simulink model "MyModel"  (R2020b)
settings: Solver=VariableStepAuto  StartTime=0.0  StopTime=50  RelTol=1e-3
undefined symbols (not defined in the file or in its folder): InnerLoop
libraries: simulink x6
settings Model: Creator=Aurelien_Julien  LastModifiedBy=Aurelien_Julien

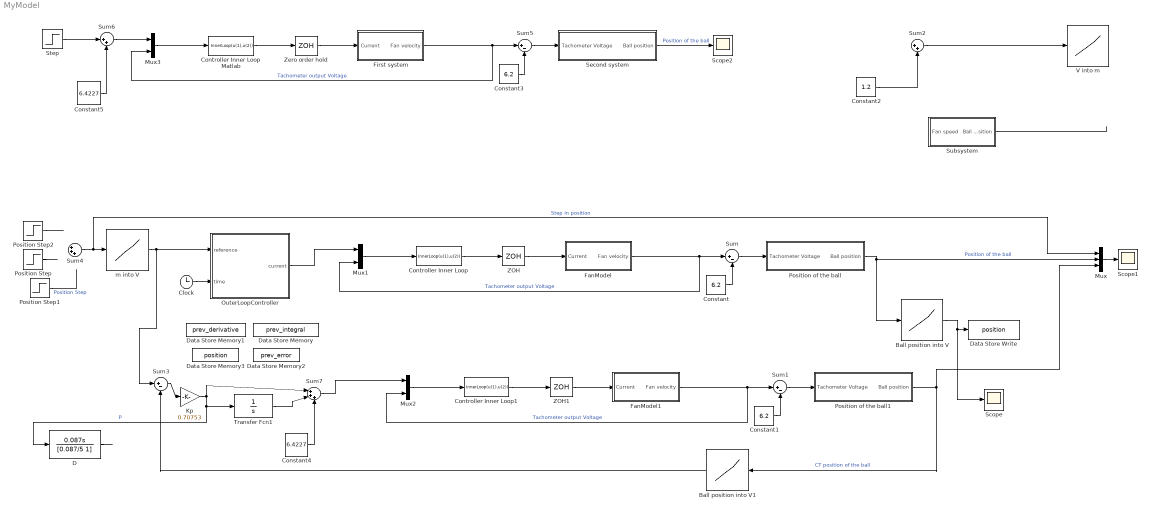
== system MyModel ==
  Ball position into V : Lookup_n-D  NumberOfTableDimensions=1  BreakpointsForDimension1=[0 15 60 97.5 117.5 125 127.5 132 135 138 142 148 152 160 167.5 180]/100  Table=[1.2 1.4 1.8 2.4 2.5 2.75 3.1 3.5 3.9 4.5 5.2 5.6 5.7 6.3 6.7 7.32]  InternalRulePriority=Speed  RndMeth=Simplest  InputSameDT=on
  Ball position into V1 : Lookup_n-D  NumberOfTableDimensions=1  BreakpointsForDimension1=[0 15 60 97.5 117.5 125 127.5 132 135 138 142 148 152 160 167.5 180]/100  Table=[1.2 1.4 1.8 2.4 2.5 2.75 3.1 3.5 3.9 4.5 5.2 5.6 5.7 6.3 6.7 7.32]  InternalRulePriority=Speed  RndMeth=Simplest  InputSameDT=on
  Clock : Clock
  Constant : Constant  Value=6.2
  Constant1 : Constant  Value=6.2
  Constant2 : Constant  Value=1.2
  Constant3 : Constant  Value=6.2
  Constant4 : Constant  Value=6.4227
  Constant5 : Constant  Value=6.4227
  Controller Inner Loop : MATLABFcn  MATLABFcn=InnerLoop(u(1),u(2))  OutputDimensions=1
  Controller Inner Loop Matlab : MATLABFcn  MATLABFcn=InnerLoop(u(1),u(2))  OutputDimensions=1
  Controller Inner Loop1 : MATLABFcn  MATLABFcn=InnerLoop(u(1),u(2))  OutputDimensions=1
  D : TransferFcn  Numerator=[0.087 0]  Denominator=[0.087/5 1]
  Data Store Memory : DataStoreMemory  DataStoreName=prev_integral  ReadBeforeWriteMsg=warning  WriteAfterWriteMsg=warning  WriteAfterReadMsg=warning  ShowAdditionalParam=off  OutDataTypeStr=double
  Data Store Memory1 : DataStoreMemory  DataStoreName=prev_derivative  ReadBeforeWriteMsg=warning  WriteAfterWriteMsg=warning  WriteAfterReadMsg=warning  ShowAdditionalParam=off  OutDataTypeStr=double
  Data Store Memory2 : DataStoreMemory  DataStoreName=prev_error  ReadBeforeWriteMsg=warning  WriteAfterWriteMsg=warning  WriteAfterReadMsg=warning  ShowAdditionalParam=off  OutDataTypeStr=double
  Data Store Memory3 : DataStoreMemory  DataStoreName=position  ReadBeforeWriteMsg=warning  WriteAfterWriteMsg=warning  WriteAfterReadMsg=warning  ShowAdditionalParam=off  OutDataTypeStr=double
  Data Store Write : DataStoreWrite  DataStoreName=position  SampleTime=0.01
  FanModel : Subsystem
  FanModel1 : Subsystem
  First system : Subsystem
  Kp : Gain  Gain=0.70753
  Mux : Mux  Inputs=3
  Mux1 : Mux  Inputs=2
  Mux2 : Mux  Inputs=2
  Mux3 : Mux  Inputs=2
  OuterLoopController : MATLAB Function  TreatAsAtomicUnit=on  SystemSampleTime=0.01
  Position Step : Step  Time=20  Before=1.2  After=1.6  SampleTime=0
  Position Step1 : Step  Time=30  After=-0.3  SampleTime=0
  Position Step2 : Step  Time=5  After=0.8  SampleTime=0
  Position of the ball : Subsystem
  Position of the ball1 : Subsystem
  Scope : Scope
  Scope1 : Scope
  Scope2 : Scope
  Second system : Subsystem
  Step : Step  SampleTime=0
  Subsystem : Subsystem
  Sum{,1,3,5} (4 alike) : Sum  Inputs=|+-
  Sum2 : Sum  Inputs=|++
  Sum4 : Sum  Inputs=|+++
  Sum6 : Sum  Inputs=|++
  Sum7 : Sum  Inputs=|+++
  Transfer Fcn1 : TransferFcn  Denominator=[1 0]
  V into m : Lookup_n-D  NumberOfTableDimensions=1  BreakpointsForDimension1=[1.2 1.4 1.8 2.4 2.5 2.75 3.1 3.5 3.9 4.5 5.2 5.6 5.7 6.3 6.7 7.32]  Table=[0 15 60 97.5 117.5 125 127.5 132 135 138 142 148 152 160 167.5 180]/100  InternalRulePriority=Speed  RndMeth=Simplest  InputSameDT=on
  ZOH : ZeroOrderHold  SampleTime=0.01
  ZOH1 : ZeroOrderHold  SampleTime=0.01
  Zero order hold : ZeroOrderHold  SampleTime=0.01
  m into V : Lookup_n-D  NumberOfTableDimensions=1  BreakpointsForDimension1=[0 15 60 97.5 117.5 125 127.5 132 135 138 142 148 152 160 167.5 180]/100  Table=[1.2 1.4 1.8 2.4 2.5 2.75 3.1 3.5 3.9 4.5 5.2 5.6 5.7 6.3 6.7 7.32]  InternalRulePriority=Speed  RndMeth=Simplest  InputSameDT=on
  wires:
  Subsystem/1(Ball Position) -> ?
  Mux1/1 -> Controller Inner Loop/1
  FanModel/1(Fan velocity) -> Sum/1, Mux1/2  "Tachometer output Voltage"
  ZOH/1 -> FanModel/1(Current)
  Controller Inner Loop/1 -> ZOH/1
  Mux/1 -> Scope1/1
  Sum/1 -> Position of the ball/1(Tachometer Voltage)
  Constant/1 -> Sum/2
  Position of the ball/1(Ball position) -> Mux/2, Ball position into V/1  "Position of the ball"
  Sum2/1 -> V into m/1
  Constant2/1 -> Sum2/2
  Sum4/1 -> Mux/1, m into V/1  "Step in position"
  Ball position into V/1 -> Scope/1, Data Store Write/1
  Kp/1 -> Transfer Fcn1/1, D/1, Sum7/1  "P"
  Constant4/1 -> Sum7/3
  Position Step1/1 -> ?  "Position Step"
  D/1 -> ?
  Clock/1 -> OuterLoopController/2(time)
  OuterLoopController/1(current) -> Mux1/1
  m into V/1 -> Sum3/1, OuterLoopController/1(reference)
  Position Step/1 -> ?
  Position Step2/1 -> ?
  Sum1/1 -> Position of the ball1/1(Tachometer Voltage)
  Constant1/1 -> Sum1/2
  FanModel1/1(Fan velocity) -> Sum1/1, Mux2/2  "Tachometer output Voltage"
  Controller Inner Loop1/1 -> ZOH1/1
  ZOH1/1 -> FanModel1/1(Current)
  Sum7/1 -> Mux2/1
  Mux2/1 -> Controller Inner Loop1/1
  Position of the ball1/1(Ball position) -> Mux/3, Ball position into V1/1  "CT position of the ball"
  Sum3/1 -> Kp/1
  Ball position into V1/1 -> Sum3/2
  Transfer Fcn1/1 -> Sum7/2
  Constant3/1 -> Sum5/2
  Sum5/1 -> Second system/1(Tachometer Voltage)
  First system/1(Fan velocity) -> Sum5/1, Mux3/2  "Tachometer output Voltage"
  Zero order hold/1 -> First system/1(Current)
  Controller Inner Loop Matlab/1 -> Zero order hold/1
  Step/1 -> Sum6/1
  Mux3/1 -> Controller Inner Loop Matlab/1
  Second system/1(Ball position) -> Scope2/1  "Position of the ball"
  Constant5/1 -> Sum6/2
  Sum6/1 -> Mux3/1

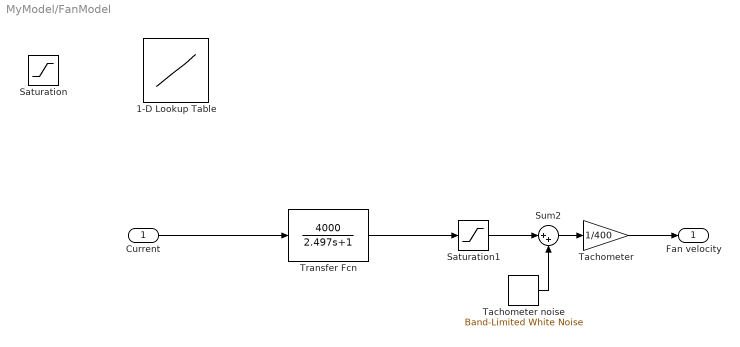
== system MyModel/FanModel ==
  Current : Inport
  1-D Lookup Table : Lookup_n-D  NumberOfTableDimensions=1  BreakpointsForDimension1=[-4 -1 0 1 2 2.5 4]  Table=[-1450 -1300 0 1600 2800 3600 3800]  InternalRulePriority=Speed  RndMeth=Simplest  InputSameDT=on
  Saturation : Saturate  UpperLimit=7  LowerLimit=-7
  Saturation1 : Saturate  UpperLimit=9.6*400  LowerLimit=-3.6*400
  Sum2 : Sum  Inputs=|++
  Tachometer : Gain  Gain=1/400
  Tachometer noise : simulink/Sources/Band-Limited White Noise  Cov=[0.1]  Ts=0.01  seed=[23341]
  Transfer Fcn : TransferFcn  Numerator=[4000]  Denominator=[2.497 1]
  Fan velocity : Outport
  wires:
  Transfer Fcn/1 -> Saturation1/1
  Current/1 -> Transfer Fcn/1
  Tachometer/1 -> Fan velocity/1
  Tachometer noise/1 -> Sum2/2
  Saturation1/1 -> Sum2/1
  Sum2/1 -> Tachometer/1

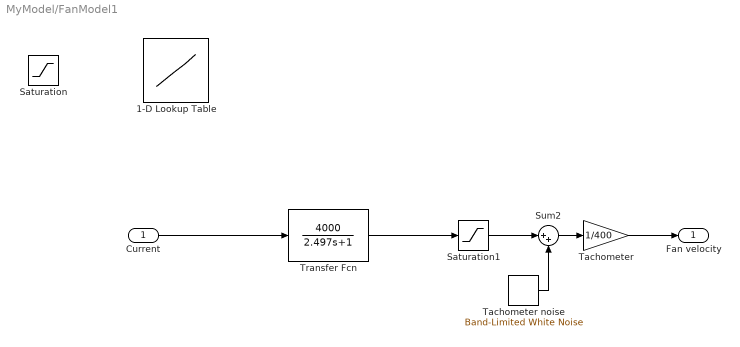
== system MyModel/FanModel1 ==
  Current : Inport
  1-D Lookup Table : Lookup_n-D  NumberOfTableDimensions=1  BreakpointsForDimension1=[-4 -1 0 1 2 2.5 4]  Table=[-1450 -1300 0 1600 2800 3600 3800]  InternalRulePriority=Speed  RndMeth=Simplest  InputSameDT=on
  Saturation : Saturate  UpperLimit=7  LowerLimit=-7
  Saturation1 : Saturate  UpperLimit=9.6*400  LowerLimit=-3.6*400
  Sum2 : Sum  Inputs=|++
  Tachometer : Gain  Gain=1/400
  Tachometer noise : simulink/Sources/Band-Limited White Noise  Cov=[0.1]  Ts=0.01  seed=[23341]
  Transfer Fcn : TransferFcn  Numerator=[4000]  Denominator=[2.497 1]
  Fan velocity : Outport
  wires:
  Transfer Fcn/1 -> Saturation1/1
  Current/1 -> Transfer Fcn/1
  Tachometer/1 -> Fan velocity/1
  Tachometer noise/1 -> Sum2/2
  Saturation1/1 -> Sum2/1
  Sum2/1 -> Tachometer/1

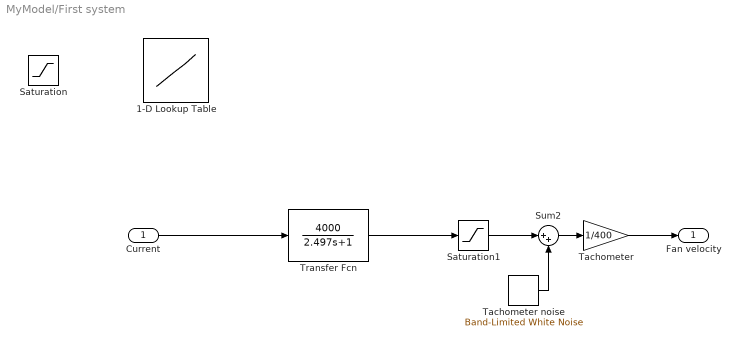
== system MyModel/First system ==
  Current : Inport
  1-D Lookup Table : Lookup_n-D  NumberOfTableDimensions=1  BreakpointsForDimension1=[-4 -1 0 1 2 2.5 4]  Table=[-1450 -1300 0 1600 2800 3600 3800]  InternalRulePriority=Speed  RndMeth=Simplest  InputSameDT=on
  Saturation : Saturate  UpperLimit=7  LowerLimit=-7
  Saturation1 : Saturate  UpperLimit=9.6*400  LowerLimit=-3.6*400
  Sum2 : Sum  Inputs=|++
  Tachometer : Gain  Gain=1/400
  Tachometer noise : simulink/Sources/Band-Limited White Noise  Cov=[0.1]  Ts=0.01  seed=[23341]
  Transfer Fcn : TransferFcn  Numerator=[4000]  Denominator=[2.497 1]
  Fan velocity : Outport
  wires:
  Transfer Fcn/1 -> Saturation1/1
  Current/1 -> Transfer Fcn/1
  Tachometer/1 -> Fan velocity/1
  Tachometer noise/1 -> Sum2/2
  Saturation1/1 -> Sum2/1
  Sum2/1 -> Tachometer/1

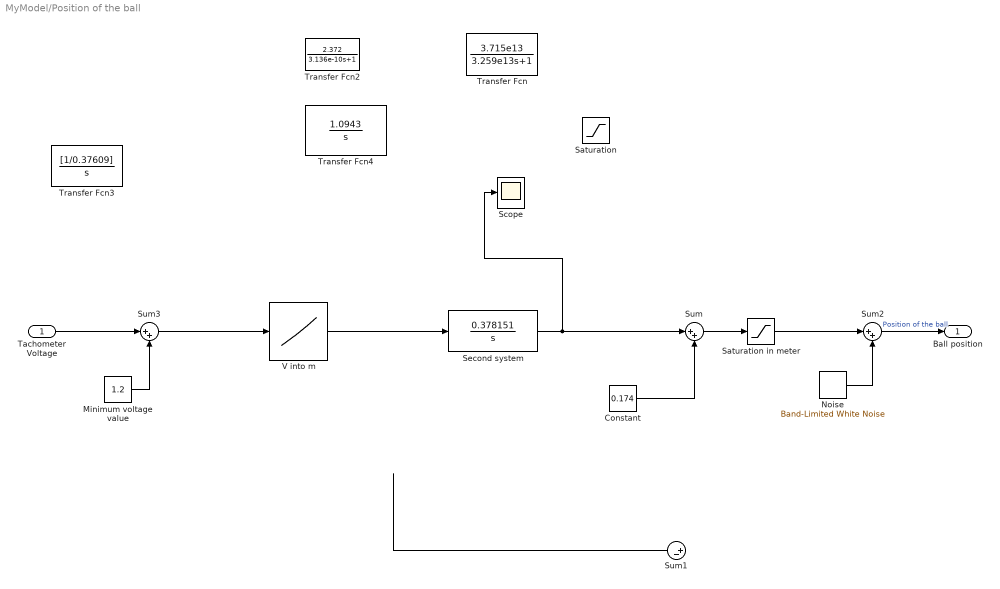
== system MyModel/Position of the ball ==
  Tachometer Voltage : Inport
  Constant : Constant  Value=0.174
  Minimum voltage value : Constant  Value=1.2
  Noise : simulink/Sources/Band-Limited White Noise  Cov=[0.0000001]  Ts=0.01  seed=[23341]
  Saturation : Saturate  UpperLimit=6.12  LowerLimit=0
  Saturation in meter : Saturate  UpperLimit=1.8  LowerLimit=0
  Scope : Scope
  Second system : TransferFcn  Numerator=[0.378151]  Denominator=[1 0]
  Sum : Sum  Inputs=|++
  Sum1 : Sum  Inputs=|+-
  Sum2 : Sum  Inputs=|++
  Sum3 : Sum  Inputs=|++
  Transfer Fcn : TransferFcn  Numerator=[3.715e13]  Denominator=[3.259e13 1]
  Transfer Fcn2 : TransferFcn  Numerator=[2.372]  Denominator=[3.136e-10 1]
  Transfer Fcn3 : TransferFcn  Numerator=[1/0.37609]  Denominator=[1 0]
  Transfer Fcn4 : TransferFcn  Numerator=[1.0943]  Denominator=[1 0]
  V into m : Lookup_n-D  NumberOfTableDimensions=1  BreakpointsForDimension1=[1.2 1.4 1.8 2.4 2.5 2.75 3.1 3.5 3.9 4.5 5.2 5.6 5.7 6.3 6.7 7.32]  Table=[0 15 60 97.5 117.5 125 127.5 132 135 138 142 148 152 160 167.5 180]/100  InternalRulePriority=Speed  RndMeth=Simplest  InputSameDT=on
  Ball position : Outport
  wires:
  Constant/1 -> Sum/2
  Sum/1 -> Saturation in meter/1
  Sum1/1 -> ?
  Minimum voltage value/1 -> Sum3/2
  Second system/1 -> Scope/1, Sum/1
  Saturation in meter/1 -> Sum2/1
  V into m/1 -> Second system/1
  Tachometer Voltage/1 -> Sum3/1
  Sum3/1 -> V into m/1
  Noise/1 -> Sum2/2
  Sum2/1 -> Ball position/1  "Position of the ball"

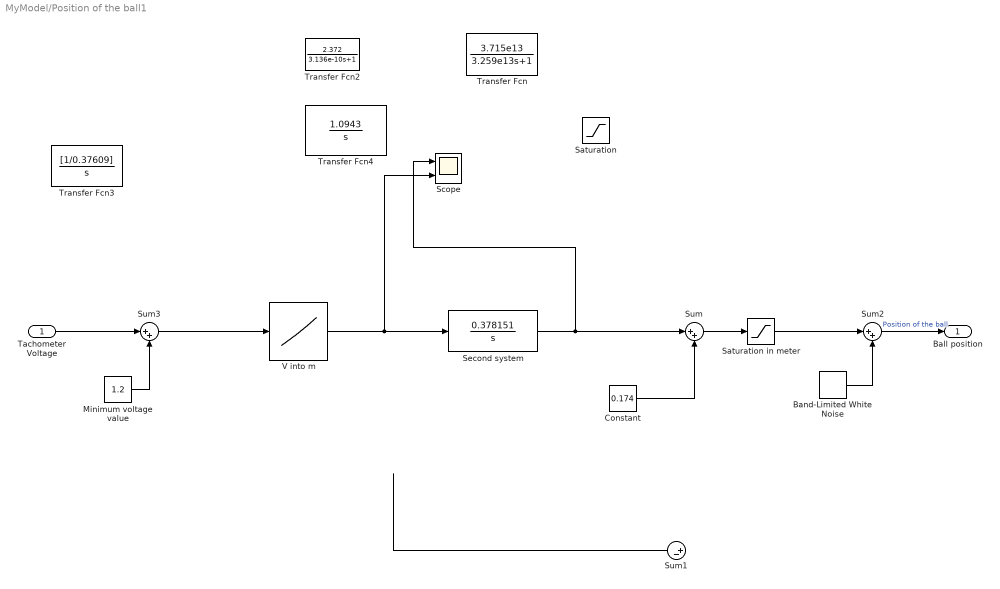
== system MyModel/Position of the ball1 ==
  Tachometer Voltage : Inport
  Band-Limited White Noise : simulink/Sources/Band-Limited White Noise  Cov=[0.0000001]  Ts=0.01  seed=[23341]
  Constant : Constant  Value=0.174
  Minimum voltage value : Constant  Value=1.2
  Saturation : Saturate  UpperLimit=6.12  LowerLimit=0
  Saturation in meter : Saturate  UpperLimit=1.8  LowerLimit=0
  Scope : Scope  NumInputPorts=2
  Second system : TransferFcn  Numerator=[0.378151]  Denominator=[1 0]
  Sum : Sum  Inputs=|++
  Sum1 : Sum  Inputs=|+-
  Sum2 : Sum  Inputs=|++
  Sum3 : Sum  Inputs=|++
  Transfer Fcn : TransferFcn  Numerator=[3.715e13]  Denominator=[3.259e13 1]
  Transfer Fcn2 : TransferFcn  Numerator=[2.372]  Denominator=[3.136e-10 1]
  Transfer Fcn3 : TransferFcn  Numerator=[1/0.37609]  Denominator=[1 0]
  Transfer Fcn4 : TransferFcn  Numerator=[1.0943]  Denominator=[1 0]
  V into m : Lookup_n-D  NumberOfTableDimensions=1  BreakpointsForDimension1=[1.2 1.4 1.8 2.4 2.5 2.75 3.1 3.5 3.9 4.5 5.2 5.6 5.7 6.3 6.7 7.32]  Table=[0 15 60 97.5 117.5 125 127.5 132 135 138 142 148 152 160 167.5 180]/100  InternalRulePriority=Speed  RndMeth=Simplest  InputSameDT=on
  Ball position : Outport
  wires:
  Constant/1 -> Sum/2
  Sum/1 -> Saturation in meter/1
  Sum1/1 -> ?
  Minimum voltage value/1 -> Sum3/2
  Second system/1 -> Scope/1, Sum/1
  Saturation in meter/1 -> Sum2/1
  V into m/1 -> Scope/2, Second system/1
  Tachometer Voltage/1 -> Sum3/1
  Sum3/1 -> V into m/1
  Band-Limited White Noise/1 -> Sum2/2
  Sum2/1 -> Ball position/1  "Position of the ball"

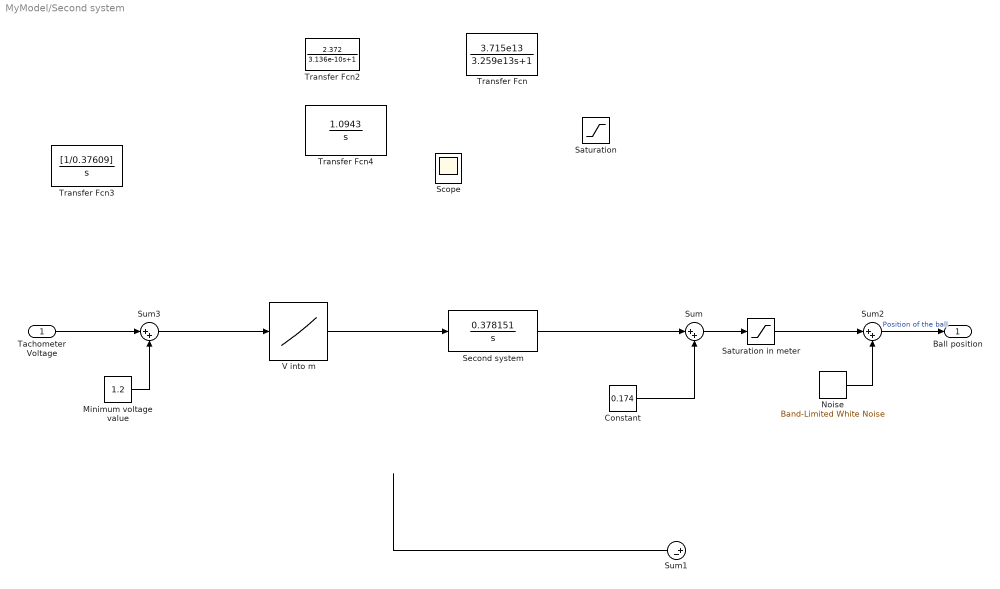
== system MyModel/Second system ==
  Tachometer Voltage : Inport
  Constant : Constant  Value=0.174
  Minimum voltage value : Constant  Value=1.2
  Noise : simulink/Sources/Band-Limited White Noise  Cov=[0.0000001]  Ts=0.01  seed=[23341]
  Saturation : Saturate  UpperLimit=6.12  LowerLimit=0
  Saturation in meter : Saturate  UpperLimit=1.8  LowerLimit=0
  Scope : Scope  NumInputPorts=2
  Second system : TransferFcn  Numerator=[0.378151]  Denominator=[1 0]
  Sum : Sum  Inputs=|++
  Sum1 : Sum  Inputs=|+-
  Sum2 : Sum  Inputs=|++
  Sum3 : Sum  Inputs=|++
  Transfer Fcn : TransferFcn  Numerator=[3.715e13]  Denominator=[3.259e13 1]
  Transfer Fcn2 : TransferFcn  Numerator=[2.372]  Denominator=[3.136e-10 1]
  Transfer Fcn3 : TransferFcn  Numerator=[1/0.37609]  Denominator=[1 0]
  Transfer Fcn4 : TransferFcn  Numerator=[1.0943]  Denominator=[1 0]
  V into m : Lookup_n-D  NumberOfTableDimensions=1  BreakpointsForDimension1=[1.2 1.4 1.8 2.4 2.5 2.75 3.1 3.5 3.9 4.5 5.2 5.6 5.7 6.3 6.7 7.32]  Table=[0 15 60 97.5 117.5 125 127.5 132 135 138 142 148 152 160 167.5 180]/100  InternalRulePriority=Speed  RndMeth=Simplest  InputSameDT=on
  Ball position : Outport
  wires:
  Constant/1 -> Sum/2
  Sum/1 -> Saturation in meter/1
  Sum1/1 -> ?
  Minimum voltage value/1 -> Sum3/2
  Second system/1 -> Sum/1
  Saturation in meter/1 -> Sum2/1
  V into m/1 -> Second system/1
  Tachometer Voltage/1 -> Sum3/1
  Sum3/1 -> V into m/1
  Noise/1 -> Sum2/2
  Sum2/1 -> Ball position/1  "Position of the ball"

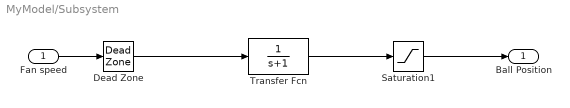
== system MyModel/Subsystem ==
  Fan speed : Inport
  Dead Zone : DeadZone  LowerValue=-11  UpperValue=6.25  SaturateOnIntegerOverflow=on
  Saturation1 : Saturate  UpperLimit=7.32  LowerLimit=1.2
  Transfer Fcn : TransferFcn  Denominator=[1 1]
  Ball Position : Outport
  wires:
  Fan speed/1 -> Dead Zone/1
  Dead Zone/1 -> Transfer Fcn/1
  Transfer Fcn/1 -> Saturation1/1
  Saturation1/1 -> Ball Position/1

== matlab function MyModel/OuterLoopController ==
  data: reference input; current output; time input; prev_integral data_store_memory; prev_derivative data_store_memory; prev_error data_store_memory; position data_store_memory
function current = OuterLoopController(reference,time)
global prev_integral;
global prev_derivative;
global prev_error;
global position;

if(time == 0)
   prev_error = 0;
   prev_integral = 0;
   prev_derivative = 0;
end

Ts = 0.01;

if (position < 2.5)
    Kp = 5.0766;
else
    Kp = 0.70753;
end

error = reference - position;
integral = 0;
derivative = prev_derivative*0.5536+3.884*error-3.884*prev_error;
current = Kp*error + Kp*integral + Kp*derivative;

prev_integral = integral;
prev_derivative = derivative;
prev_error = error;

current = current + 6.4227;

if(abs(current)>10)
    current = 10*sign(current);
end

end
